simulink subsystem "s0330_alpha_theta_LQ_up"  (R2019b)
settings: Solver=VariableStepAuto  StartTime=0.0  StopTime=10.0  RelTol=1e-3
undefined symbols (not defined in the file): __PRM__SERIALIZED__DATA__, PARAMS, SubsystemReferenceBlock
settings Model: Creator=francescoceresetti  LastModifiedBy=giaco

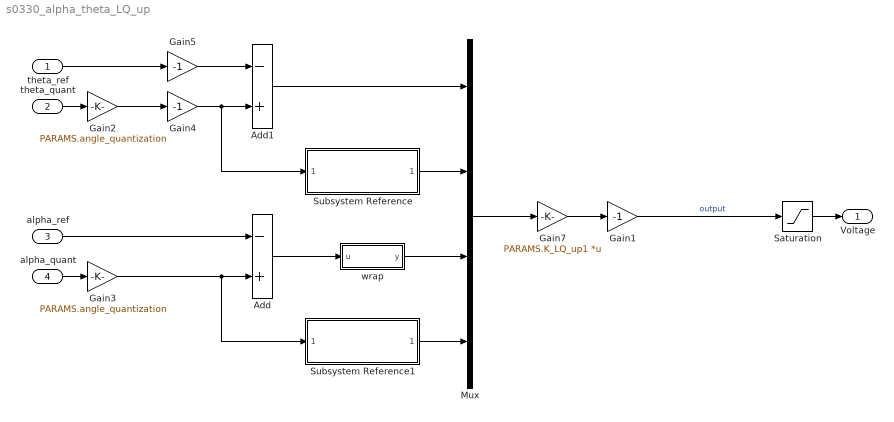
== system s0330_alpha_theta_LQ_up ==
  theta_ref : Inport
  theta_quant : Inport  Port=2
  alpha_ref : Inport  Port=3
  alpha_quant : Inport  Port=4
  Add : Sum  Inputs=-+
  Add1 : Sum  Inputs=-+
  Gain1 : Gain  Gain=-1
  Gain2 : Gain  Gain=PARAMS.angle_quantization
  Gain3 : Gain  Gain=PARAMS.angle_quantization
  Gain4 : Gain  Gain=-1
  Gain5 : Gain  Gain=-1
  Gain7 : Gain  Gain=PARAMS.K_LQ_up1  Multiplication=Matrix(K*u)
  Mux : Mux
  Saturation : Saturate  UpperLimit=PARAMS.V_sat  LowerLimit=-PARAMS.V_sat
  Subsystem Reference : Subsystem  BlockKeywords=__PRM__SERIALIZED__DATA__:SubsystemReferenceBlock  ReferencedSubsystem=Filtered_Derivative  num=num_der_filter  den=den_der_filter
  Subsystem Reference1 : Subsystem  BlockKeywords=__PRM__SERIALIZED__DATA__:SubsystemReferenceBlock  ReferencedSubsystem=Filtered_Derivative  num=num_der_filter  den=den_der_filter
  wrap : MATLAB Function  TreatAsAtomicUnit=on
  Voltage : Outport
  wires:
  alpha_quant/1 -> Gain3/1
  Mux/1 -> Gain7/1
  Gain7/1 -> Gain1/1
  Add1/1 -> Mux/1
  theta_quant/1 -> Gain2/1
  alpha_ref/1 -> Add/1
  Add/1 -> wrap/1(u)
  wrap/1(y) -> Mux/3
  Saturation/1 -> Voltage/1
  Gain4/1 -> Add1/2, Subsystem Reference/1
  Gain5/1 -> Add1/1
  theta_ref/1 -> Gain5/1
  Gain2/1 -> Gain4/1
  Gain3/1 -> Add/2, Subsystem Reference1/1
  Gain1/1 -> Saturation/1  "output"
  Subsystem Reference/1 -> Mux/2
  Subsystem Reference1/1 -> Mux/4

== matlab function s0330_alpha_theta_LQ_up/wrap ==
  data: u input; y output
function y = wrap(u)
stop_condition = false;
y = u;
while ~stop_condition
    if y > pi
        y = y - 2*pi;
    elseif y < -pi
        y = y + 2*pi;
    else
        stop_condition = true;
    end
end
